simulink library "Simple_House"  (Simulink 8.2)
settings: Solver=ode45  StartTime=0.0  StopTime=10.0  RelTol=1e-3
libraries: carnot x4
settings Model: Creator=lena.frank  LastModifiedBy=drhf

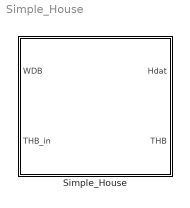
== system Simple_House ==
  Simple_House : Subsystem  mask(simple house){Ahabit=30, Hroom=2.5, Floorsize=[5 6], UAwall=0.162*(30)+0.182*((5+6)*2*2.5 -(4+0+0+0)), UAneighbour=0, Uground=0  %0.18 wenn Wert verlangt, mc=0.5e6*30   % 0.5 MJ/m2/K, shade=0.75, tini=20, Awin=[4 0 0 0], AziWin=[0 90 -180 -90], Uwin=[1    1   1    1]*1.5, Gwin=[1    1   1    1]*0.7*(1-0.15), vent=0.4, rec=0, heatload=2000, dpcoeff=[10 100], delta_t_nom=50, n_rad=1.1, mass_times_cap=40e6}
      mask prompts: Ahabit "Living surface in m²"; Hroom "height of rooms in m"; Floorsize "Dimensions of slab in m [length width]"; UAwall "Total heat transfer to ambient (walls/roof) in W/K"; UAneighbour "Total heat transfer to neighbour inW/K"; Uground "Heat transfer coeffient to ground in W/m²/K"; mc "Total thermal capacity in J/K"; shade "Shading factor [0..1] when T room > 4 K + T_init"; tini "Initial temperature"; Awin "Surface of 4 windows in m² (vector)"; AziWin "Orientation of 4 windows (south 0, east -90,west 90)"; Uwin "Heat loss coefficient 4 windows in W/m²/K [vector]"; Gwin "Light transmittance 4 windows (0..1) * (1 - frame_part) [vector]"; vent "Ventilation rate in 1/h"; rec "Heat recovery (0..1)"; heatload "Heating capacity radiator  [W]"; dpcoeff "Pressure drop coefficients [linear quadratic] in Pa/(kg/s), Pa/(kg/s)²"; delta_t_nom "Nominal delta T (average radiator temperature - room temperature) [K]"; n_rad "Radiator exponent"; mass_times_cap "Mass*capacity of heating system [J/K]"
      mask help:
      | Simple model of 1-node room or house. The differential equation
      | (m*c)house * dT/dt = solar_gain + internal_gain + heating_power - losses_to_ambient - losses_to_neighbour_room
      | is solved.
      | The heating power is generated by a radiator or floor heating system.
      | The windows have an automatic shading (shading factor) if room temperature rises 4 K above initial temperature.
      | solar gain = Solar_Radiation_on_window * light_transmittance * shading_factor
      | Use "look under mask" to set up the models parameters (initial conditions, surfaces characteristics...).
      | A usual value for the internal gains is 2.3 W/m².
      mask init:
      | invmc = 1/mc;
      | rec = max(0,min(1,rec));
      | Gwin = max(0,min(1,Gwin));
      | shade = max(0, min(1, shade));
      mask Help: web(fullfile(path_carnot('help'),'simple_house.html'),'-helpbrowser')
      mask Display: plot(0,-15,80,100,[30,30,60,60,30],[20,50,50,20,20],[47,47,56,56,47],[40,30,30,40,40],[42,42,34,34],[20,40,40,20],[62,45,28],[48,70,48])

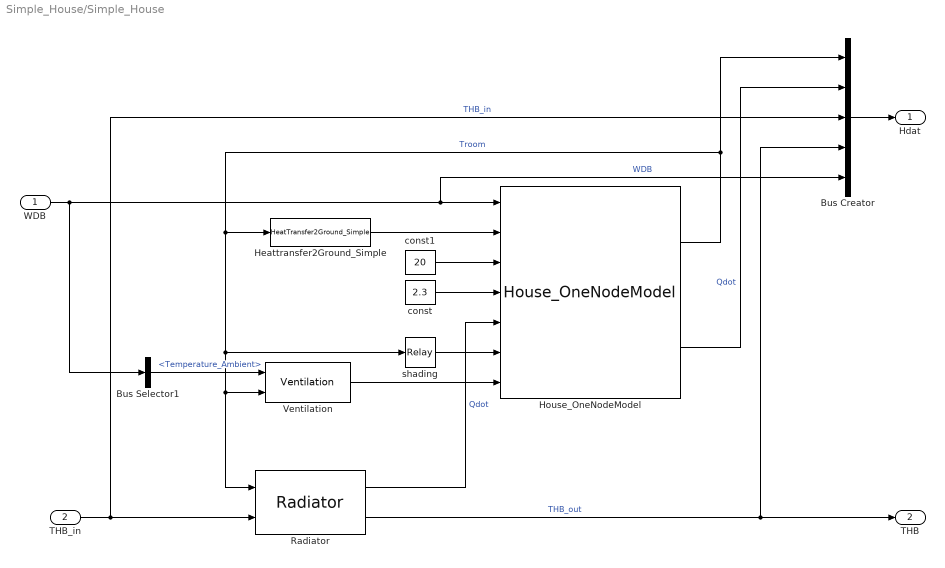
== system Simple_House/Simple_House ==
  WDB : Inport
  THB_in : Inport  Port=2
  Bus Creator : BusCreator  Inputs=5
  Bus Selector1 : BusSelector  OutputSignals=Temperature_Ambient
  Heattransfer2Ground_Simple : carnot/Load/Houses/heat_transfer/HeatTransfer2Ground_Simple  Tground=10  UAground=Uground*Floorsize(1)*Floorsize(2)
  House_OneNodeModel : carnot/Basic/Thermal_Models/House_OneNodeModel  Ahabit=Ahabit  Hroom=Hroom  tini=tini  UAout=UAwall  mc=mc  UAin=UAneighbour  dtroom=inf  AziWin=AziWin  Awin=Awin  Uwin=Uwin  Gwin=Gwin
  Radiator : carnot/Source/Heat_Exchanger/Radiator  pnom=heatload  dtnom=delta_t_nom  expo=n_rad  mcap=mass_times_cap  tini=tini  lin=0  qua=1000
  Ventilation : carnot/Source/Ventilation/Ventilation  vent=vent  rec=rec  Vhouse=Ahabit*Hroom
  const : Constant  Value=2.3
  const1 : Constant  Value=20
  shading : Relay  OnSwitchValue=24  OffSwitchValue=23  OnOutputValue=1-shade  OffOutputValue=1
  Hdat : Outport
  THB : Outport  Port=2
  wires:
  Bus Selector1/1 -> Ventilation/1  "<Temperature_Ambient>"
  Heattransfer2Ground_Simple/1 -> House_OneNodeModel/2
  Radiator/1 -> House_OneNodeModel/5  "Qdot"
  Radiator/2 -> THB/1, Bus Creator/4  "THB_out"
  House_OneNodeModel/1 -> Heattransfer2Ground_Simple/1, Ventilation/2, Radiator/1, shading/1, Bus Creator/1  "Troom"
  THB_in/1 -> Radiator/2, Bus Creator/3  "THB_in"
  WDB/1 -> House_OneNodeModel/1, Bus Creator/5, Bus Selector1/1  "WDB"
  Bus Creator/1 -> Hdat/1
  const1/1 -> House_OneNodeModel/3
  House_OneNodeModel/2 -> Bus Creator/2  "Qdot"
  shading/1 -> House_OneNodeModel/6
  const/1 -> House_OneNodeModel/4
  Ventilation/1 -> House_OneNodeModel/7
